simulink model "Newton_Euler_RP_LATEST"  (R2023b)
settings: Solver=VariableStepAuto  StartTime=0.0  StopTime=20  RelTol=1e-3
undefined symbols (not defined in the file or in its folder): L11, L22, M1, M2, X, Y, Z
libraries: nesl_utility x25, sm_lib x20, robotcorelib x1, simulink x1
settings Model: Creator=manu  LastModifiedBy=hdelala
settings DebuggingCC: UnconnectedInputMsg=warning  UnconnectedOutputMsg=warning  UnconnectedLineMsg=warning
settings ModelReferenceCC: EnableRefExpFcnMdlSchedulingChecks=on
settings RTWCC: DLArmComputeVersion=19.05

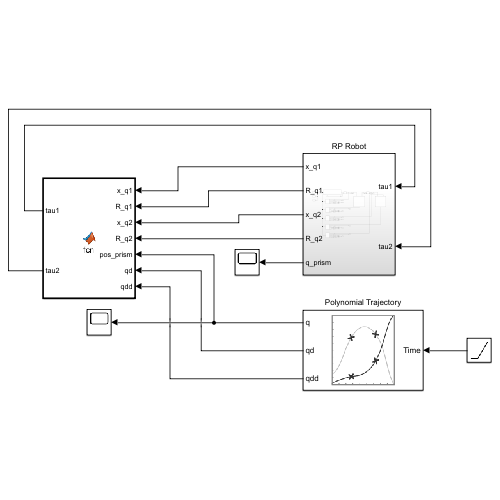
[thumbnail: Simulink's stored preview of the top-level diagram]
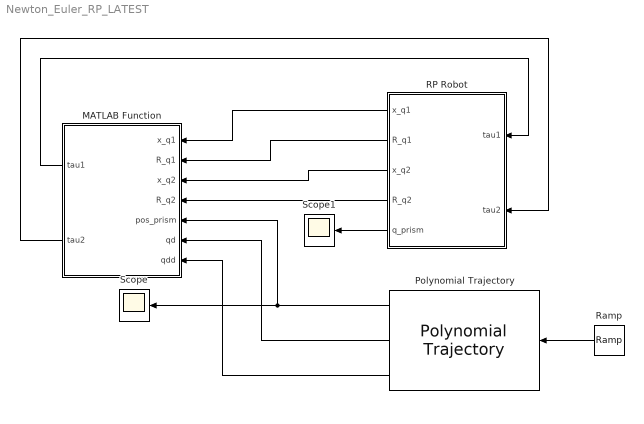
== system Newton_Euler_RP_LATEST ==
  MATLAB Function : MATLAB Function  TreatAsAtomicUnit=on
  Polynomial Trajectory : robotcorelib/Polynomial Trajectory  WaypointSource=Internal  Waypoints=[0,pi/4;-5/100,-10/100]  TimePoints=[ 0, 15 ]  TimeInterval=[ 1, 4 ]  Method=Cubic Polynomial  ParameterSource=Internal  VelocityBoundaryCondition=zeros( 2, 2 )  AccelerationBoundaryCondition=zeros( 2, 5 )  SimulateUsing=Interpreted execution
  RP Robot : Subsystem
  Ramp : simulink/Sources/Ramp  slope=1  start=0  InitialOutput=0
  Scope : Scope
  Scope1 : Scope
  wires:
  Polynomial Trajectory/1 -> MATLAB Function/5(pos_prism), Scope/1
  Ramp/1 -> Polynomial Trajectory/1
  MATLAB Function/2(tau2) -> RP Robot/2(tau2)
  MATLAB Function/1(tau1) -> RP Robot/1(tau1)
  RP Robot/1(x_q1) -> MATLAB Function/1(x_q1)
  RP Robot/2(R_q1) -> MATLAB Function/2(R_q1)
  RP Robot/3(x_q2) -> MATLAB Function/3(x_q2)
  RP Robot/4(R_q2) -> MATLAB Function/4(R_q2)
  Polynomial Trajectory/2 -> MATLAB Function/6(qd)
  Polynomial Trajectory/3 -> MATLAB Function/7(qdd)
  RP Robot/5(q_prism) -> Scope1/1

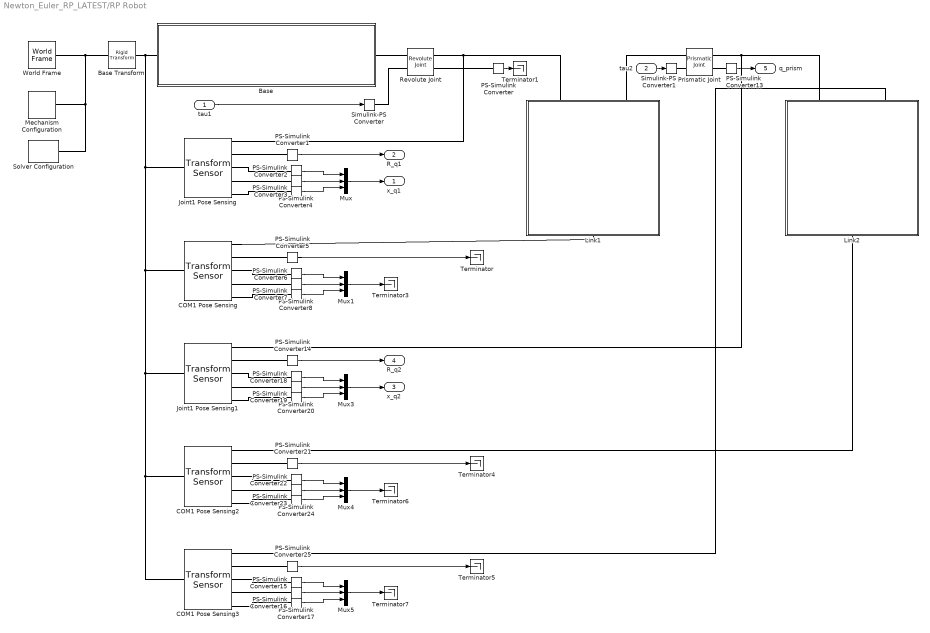
== system Newton_Euler_RP_LATEST/RP Robot ==
  tau1 : Inport
  tau2 : Inport  Port=2
  Base : Subsystem
  Base Transform : sm_lib/Frames and Transforms/Rigid Transform  TranslationMethod=None  TranslationStandardOffset=0  TranslationStandardOffsetUnits=m  TranslationStandardAxis=+Z  TranslationCartesianOffset=[0 0 0]  TranslationCartesianOffsetUnits=m  TranslationROffset=0  TranslationROffsetUnits=m  TranslationZOffset=0  TranslationZOffsetUnits=m  TranslationThetaOffset=0  TranslationThetaOffsetUnits=deg  RotationMethod=AlignedAxes  RotationAngleUnits=deg  RotationStandardAxis=+Z  RotationAngle=0.0  RotationArbitraryAxis=[0 0 1]  FollAlignAxisA=+Z  BaseAlignAxisA=-Y  FollAlignAxisB=+X  BaseAlignAxisB=+X  RotationSequenceAxes=FollowerAxes  RotationSequence=XYX  RotationSequenceAngles=[0 0 0]  RotationSequenceAnglesUnits=deg  RotationMatrix=[1 0 0; 0 1 0; 0 0 1]  Quaternion=[1 0 0 0]
  COM1 Pose Sensing : sm_lib/Frames and Transforms/Transform Sensor  MeasurementFrame=Base  RotationSequence=XYX  SenseAngle=off  SenseAxis=off  SenseQ=off  SenseR=on  SenseRotationSequence=off  SenseOmegaX=off  SenseOmegaY=off  SenseOmegaZ=off  SenseOmega=off  SenseQDot=off  SenseRDot=off  SenseRotationSequenceDot=off  SenseAlphaX=off  SenseAlphaY=off  SenseAlphaZ=off  SenseAlpha=off  SenseQDDot=off  SenseRDDot=off  SenseX=on  SenseY=on  SenseZ=on  SenseXYZ=off  SenseRad=off  SenseAzim=off  SenseDist=off  SenseInc=off  SenseXDot=off  SenseYDot=off  SenseZDot=off  SenseXYZDot=off  SenseRadDot=off  SenseAzimDot=off  SenseDistDot=off  SenseIncDot=off  SenseXDDot=off  SenseYDDot=off  SenseZDDot=off  SenseXYZDDot=off  SenseRadDDot=off  SenseAzimDDot=off  SenseDistDDot=off  SenseIncDDot=off
  COM1 Pose Sensing2 : sm_lib/Frames and Transforms/Transform Sensor  MeasurementFrame=Base  RotationSequence=XYX  SenseAngle=off  SenseAxis=off  SenseQ=off  SenseR=on  SenseRotationSequence=off  SenseOmegaX=off  SenseOmegaY=off  SenseOmegaZ=off  SenseOmega=off  SenseQDot=off  SenseRDot=off  SenseRotationSequenceDot=off  SenseAlphaX=off  SenseAlphaY=off  SenseAlphaZ=off  SenseAlpha=off  SenseQDDot=off  SenseRDDot=off  SenseX=on  SenseY=on  SenseZ=on  SenseXYZ=off  SenseRad=off  SenseAzim=off  SenseDist=off  SenseInc=off  SenseXDot=off  SenseYDot=off  SenseZDot=off  SenseXYZDot=off  SenseRadDot=off  SenseAzimDot=off  SenseDistDot=off  SenseIncDot=off  SenseXDDot=off  SenseYDDot=off  SenseZDDot=off  SenseXYZDDot=off  SenseRadDDot=off  SenseAzimDDot=off  SenseDistDDot=off  SenseIncDDot=off
  COM1 Pose Sensing3 : sm_lib/Frames and Transforms/Transform Sensor  MeasurementFrame=Base  RotationSequence=XYX  SenseAngle=off  SenseAxis=off  SenseQ=off  SenseR=on  SenseRotationSequence=off  SenseOmegaX=off  SenseOmegaY=off  SenseOmegaZ=off  SenseOmega=off  SenseQDot=off  SenseRDot=off  SenseRotationSequenceDot=off  SenseAlphaX=off  SenseAlphaY=off  SenseAlphaZ=off  SenseAlpha=off  SenseQDDot=off  SenseRDDot=off  SenseX=on  SenseY=on  SenseZ=on  SenseXYZ=off  SenseRad=off  SenseAzim=off  SenseDist=off  SenseInc=off  SenseXDot=off  SenseYDot=off  SenseZDot=off  SenseXYZDot=off  SenseRadDot=off  SenseAzimDot=off  SenseDistDot=off  SenseIncDot=off  SenseXDDot=off  SenseYDDot=off  SenseZDDot=off  SenseXYZDDot=off  SenseRadDDot=off  SenseAzimDDot=off  SenseDistDDot=off  SenseIncDDot=off
  Joint1 Pose Sensing : sm_lib/Frames and Transforms/Transform Sensor  MeasurementFrame=Base  RotationSequence=XYX  SenseAngle=off  SenseAxis=off  SenseQ=off  SenseR=on  SenseRotationSequence=off  SenseOmegaX=off  SenseOmegaY=off  SenseOmegaZ=off  SenseOmega=off  SenseQDot=off  SenseRDot=off  SenseRotationSequenceDot=off  SenseAlphaX=off  SenseAlphaY=off  SenseAlphaZ=off  SenseAlpha=off  SenseQDDot=off  SenseRDDot=off  SenseX=on  SenseY=on  SenseZ=on  SenseXYZ=off  SenseRad=off  SenseAzim=off  SenseDist=off  SenseInc=off  SenseXDot=off  SenseYDot=off  SenseZDot=off  SenseXYZDot=off  SenseRadDot=off  SenseAzimDot=off  SenseDistDot=off  SenseIncDot=off  SenseXDDot=off  SenseYDDot=off  SenseZDDot=off  SenseXYZDDot=off  SenseRadDDot=off  SenseAzimDDot=off  SenseDistDDot=off  SenseIncDDot=off
  Joint1 Pose Sensing1 : sm_lib/Frames and Transforms/Transform Sensor  MeasurementFrame=Base  RotationSequence=XYX  SenseAngle=off  SenseAxis=off  SenseQ=off  SenseR=on  SenseRotationSequence=off  SenseOmegaX=off  SenseOmegaY=off  SenseOmegaZ=off  SenseOmega=off  SenseQDot=off  SenseRDot=off  SenseRotationSequenceDot=off  SenseAlphaX=off  SenseAlphaY=off  SenseAlphaZ=off  SenseAlpha=off  SenseQDDot=off  SenseRDDot=off  SenseX=on  SenseY=on  SenseZ=on  SenseXYZ=off  SenseRad=off  SenseAzim=off  SenseDist=off  SenseInc=off  SenseXDot=off  SenseYDot=off  SenseZDot=off  SenseXYZDot=off  SenseRadDot=off  SenseAzimDot=off  SenseDistDot=off  SenseIncDot=off  SenseXDDot=off  SenseYDDot=off  SenseZDDot=off  SenseXYZDDot=off  SenseRadDDot=off  SenseAzimDDot=off  SenseDistDDot=off  SenseIncDDot=off
  Link1 : Subsystem
  Link2 : Subsystem
  Mechanism Configuration : sm_lib/Utilities/Mechanism Configuration  UniformGravity=Constant  GravityVector=[0 0 -9.81]  GravityVectorUnits=m/s^2  LinearizationDelta=0.001  JointModeTransitionNonlinearIterations=2
  Mux{,1,3..5} (5 alike) : Mux  Inputs=3
  PS-Simulink Converter{,1..8,13..25} (22 alike) : nesl_utility/PS-Simulink Converter  PhysicalDomain=network_engine_domain  SubClassName=ps_output  LeftPortType=input  RightPortType=output  PseudoPeriodic=off  Frequencies=[]  VectorFormat=1-D array  Unit=inherit  AffineConversion=off
  Prismatic Joint : sm_lib/Joints/Prismatic Joint  JointMode=Normal  SenseConstraintForce=off  SenseConstraintForceX=off  SenseConstraintForceY=off  SenseConstraintForceZ=off  SenseConstraintTorque=off  SenseConstraintTorqueX=off  SenseConstraintTorqueY=off  SenseConstraintTorqueZ=off  SenseTotalForce=off  SenseTotalForceX=off  SenseTotalForceY=off  SenseTotalForceZ=off  SenseTotalTorque=off  SenseTotalTorqueX=off  SenseTotalTorqueY=off  SenseTotalTorqueZ=off  CompositeWrenchDir=FollowerOnBase  CompositeWrenchFrame=BaseFrame  EquilibriumPosition=0  EquilibriumPositionUnits=m  SpringStiffness=0  SpringStiffnessUnits=N/m  DampingCoefficient=0  DampingCoefficientUnits=N/(m/s)  TorqueActuationMode=InputTorque  MotionActuationMode=ComputedMotion  SensePosition=on  SenseVelocity=off  SenseAcceleration=off  SenseTorqueForce=off  SenseLowerLimitTorqueForce=off  SenseUpperLimitTorqueForce=off  LowerLimitSpecify=off  LowerLimitBound=-25/2  LowerLimitBoundUnits=cm  LowerLimitStiffness=1e6  LowerLimitStiffnessUnits=N/m  LowerLimitDamping=1e3  LowerLimitDampingUnits=N/(m/s)  LowerLimitTransitionRegionWidth=1e-4  LowerLimitTransitionRegionWidthUnits=m  UpperLimitSpecify=off  UpperLimitBound=0  UpperLimitBoundUnits=cm  UpperLimitStiffness=1e6  UpperLimitStiffnessUnits=N/m  UpperLimitDamping=1e3  UpperLimitDampingUnits=N/(m/s)  UpperLimitTransitionRegionWidth=1e-4  UpperLimitTransitionRegionWidthUnits=m  PositionTargetSpecify=on  PositionTargetPriority=High  PositionTargetValue=Q2  PositionTargetValueUnits=cm  VelocityTargetSpecify=off  VelocityTargetPriority=High  VelocityTargetValue=0  VelocityTargetValueUnits=m/s
  Revolute Joint : sm_lib/Joints/Revolute Joint  JointMode=Normal  SenseConstraintForce=off  SenseConstraintForceX=off  SenseConstraintForceY=off  SenseConstraintForceZ=off  SenseConstraintTorque=off  SenseConstraintTorqueX=off  SenseConstraintTorqueY=off  SenseConstraintTorqueZ=off  SenseTotalForce=off  SenseTotalForceX=off  SenseTotalForceY=off  SenseTotalForceZ=off  SenseTotalTorque=off  SenseTotalTorqueX=off  SenseTotalTorqueY=off  SenseTotalTorqueZ=off  CompositeWrenchDir=FollowerOnBase  CompositeWrenchFrame=BaseFrame  EquilibriumPosition=0  EquilibriumPositionUnits=rad  SpringStiffness=0  SpringStiffnessUnits=N*m/rad  DampingCoefficient=0.002  DampingCoefficientUnits=N*m/(rad/s)  TorqueActuationMode=InputTorque  MotionActuationMode=ComputedMotion  SensePosition=on  SenseVelocity=off  SenseAcceleration=off  SenseTorqueForce=off  SenseLowerLimitTorqueForce=off  SenseUpperLimitTorqueForce=off  LowerLimitSpecify=off  LowerLimitBound=-90  LowerLimitBoundUnits=deg  LowerLimitStiffness=1e4  LowerLimitStiffnessUnits=N*m/deg  LowerLimitDamping=10  LowerLimitDampingUnits=N*m/(deg/s)  LowerLimitTransitionRegionWidth=0.1  LowerLimitTransitionRegionWidthUnits=deg  UpperLimitSpecify=off  UpperLimitBound=90  UpperLimitBoundUnits=deg  UpperLimitStiffness=1e4  UpperLimitStiffnessUnits=N*m/deg  UpperLimitDamping=10  UpperLimitDampingUnits=N*m/(deg/s)  UpperLimitTransitionRegionWidth=0.1  UpperLimitTransitionRegionWidthUnits=deg  PositionTargetSpecify=on  PositionTargetPriority=High  PositionTargetValue=Q1  PositionTargetValueUnits=deg  VelocityTargetSpecify=off  VelocityTargetPriority=High  VelocityTargetValue=0  VelocityTargetValueUnits=deg/s
  Simulink-PS Converter : nesl_utility/Simulink-PS Converter  PhysicalDomain=network_engine_domain  SubClassName=ps_input  LeftPortType=input  RightPortType=output  PseudoPeriodic=off  Frequencies=[]  NoiseDistribution=none  NoiseParameters=[]  Unit=1  AffineConversion=off  FilteringAndDerivatives=provide  SimscapeFilterOrder=1  InputFilterTimeConstant=0.001  UdotUserProvided=0
  Simulink-PS Converter1 : nesl_utility/Simulink-PS Converter  PhysicalDomain=network_engine_domain  SubClassName=ps_input  LeftPortType=input  RightPortType=output  PseudoPeriodic=off  Frequencies=[]  NoiseDistribution=none  NoiseParameters=[]  Unit=1  AffineConversion=off  FilteringAndDerivatives=provide  SimscapeFilterOrder=1  InputFilterTimeConstant=0.001  UdotUserProvided=0
  Solver Configuration : nesl_utility/Solver Configuration  PhysicalDomain=network_engine_domain  SubClassName=solver  LeftPortType=input  RightPortType=generic  Tones=[]  Harmonics=[]  SimulateNoise=off  Profile=off  UseLocalSampling=off  EnableSwitchedLinearOptims=on  FrequencyDomain=off  UseCCode=off  RelTol=0.001  AbsTol=1e-06  MinStep=1e-09  ToWorkspace=off  RevertToSquareIcSolve=off  NumHomotopyIterations=100  PhasorMode=off  PhasorModeNumHarmonics=1  ConsistencySolver=NEWTON_FTOL  IndexReductionMethod=DerivativeReplacement  DoDC=off  ResidualTolerance=1e-09  ConsistencyTolSource=GLOBAL  ConsistencyAbsTol=0.001  ConsistencyRelTol=0.001  ConsistencyTolFactor=0.001  UseLocalSolver=off  LocalSolverChoice=NE_BACKWARD_EULER_ADVANCER  ResolveIndetEquations=on  FunctionEvalNumThread=1  LocalSolverSampleTime=0.001  DoFixedCost=off  MaxNonlinIter=3  MaxModeIter=2  ComputeImpulses=off  ImpulseIterations=2  LinearAlgebra=Sparse  LinearAlgebraNumThread=0  EquationFormulation=NE_TIME_EF  DelaysMemoryBudget=1024  AutomaticFiltering=on  FilteringTimeConstant=0.001  PartitionStorageMethod=AS_NEEDED  PartitionMemoryBudget=1024  PartitionMethod=ROBUST  MultibodyUseLocalSolver=off  MultibodyLocalSolverChoice=ODE1  MultibodyLocalSolverSampleTime=0.001
  Terminator{,1,3..7} (7 alike) : Terminator
  World Frame : sm_lib/Frames and Transforms/World Frame
  x_q1 : Outport
  R_q1 : Outport  Port=2
  x_q2 : Outport  Port=3
  R_q2 : Outport  Port=4
  q_prism : Outport  Port=5
  wires:
  PS-Simulink Converter5/1 -> Terminator/1
  Mux1/1 -> Terminator3/1
  PS-Simulink Converter8/1 -> Mux1/2
  PS-Simulink Converter7/1 -> Mux1/3
  PS-Simulink Converter1/1 -> R_q1/1
  PS-Simulink Converter6/1 -> Mux1/1
  PS-Simulink Converter/1 -> Terminator1/1
  PS-Simulink Converter3/1 -> Mux/3
  Mux/1 -> x_q1/1
  tau1/1 -> Simulink-PS Converter/1
  PS-Simulink Converter2/1 -> Mux/1
  PS-Simulink Converter4/1 -> Mux/2
  tau2/1 -> Simulink-PS Converter1/1
  PS-Simulink Converter13/1 -> q_prism/1
  PS-Simulink Converter25/1 -> Terminator5/1
  PS-Simulink Converter15/1 -> Mux5/1
  PS-Simulink Converter17/1 -> Mux5/2
  PS-Simulink Converter16/1 -> Mux5/3
  Mux3/1 -> x_q2/1
  PS-Simulink Converter18/1 -> Mux3/1
  Mux4/1 -> Terminator6/1
  PS-Simulink Converter20/1 -> Mux3/2
  Mux5/1 -> Terminator7/1
  PS-Simulink Converter21/1 -> Terminator4/1
  PS-Simulink Converter23/1 -> Mux4/3
  PS-Simulink Converter14/1 -> R_q2/1
  PS-Simulink Converter24/1 -> Mux4/2
  PS-Simulink Converter19/1 -> Mux3/3
  PS-Simulink Converter22/1 -> Mux4/1
  connections:
  Revolute Joint/RConn2 -- PS-Simulink Converter/LConn1
  Revolute Joint/LConn1 -- Base/RConn1
  COM1 Pose Sensing/RConn4 -- PS-Simulink Converter8/LConn1
  COM1 Pose Sensing/RConn3 -- PS-Simulink Converter6/LConn1
  COM1 Pose Sensing/RConn2 -- PS-Simulink Converter5/LConn1
  Joint1 Pose Sensing1/LConn1 -- COM1 Pose Sensing3/LConn1 -- COM1 Pose Sensing2/LConn1 -- COM1 Pose Sensing/LConn1 -- Joint1 Pose Sensing/LConn1 -- Base Transform/RConn1 -- Base/LConn1
  PS-Simulink Converter1/LConn1 -- Joint1 Pose Sensing/RConn2
  PS-Simulink Converter3/LConn1 -- Joint1 Pose Sensing/RConn5
  Link1/LConn1 -- Joint1 Pose Sensing/RConn1 -- Revolute Joint/RConn1
  Mechanism Configuration/RConn1 -- Base Transform/LConn1 -- World Frame/RConn1 -- Solver Configuration/RConn1
  PS-Simulink Converter4/LConn1 -- Joint1 Pose Sensing/RConn4
  COM1 Pose Sensing/RConn5 -- PS-Simulink Converter7/LConn1
  Simulink-PS Converter/RConn1 -- Revolute Joint/LConn2
  Joint1 Pose Sensing/RConn3 -- PS-Simulink Converter2/LConn1
  COM1 Pose Sensing/RConn1 -- Link1/RConn1
  Link1/LConn2 -- Prismatic Joint/LConn1
  Joint1 Pose Sensing1/RConn1 -- Prismatic Joint/RConn1 -- Link2/LConn1
  Prismatic Joint/LConn2 -- Simulink-PS Converter1/RConn1
  Prismatic Joint/RConn2 -- PS-Simulink Converter13/LConn1
  COM1 Pose Sensing3/RConn5 -- PS-Simulink Converter16/LConn1
  PS-Simulink Converter19/LConn1 -- Joint1 Pose Sensing1/RConn5
  COM1 Pose Sensing3/RConn2 -- PS-Simulink Converter25/LConn1
  COM1 Pose Sensing3/RConn3 -- PS-Simulink Converter15/LConn1
  PS-Simulink Converter20/LConn1 -- Joint1 Pose Sensing1/RConn4
  Joint1 Pose Sensing1/RConn3 -- PS-Simulink Converter18/LConn1
  PS-Simulink Converter14/LConn1 -- Joint1 Pose Sensing1/RConn2
  COM1 Pose Sensing2/RConn2 -- PS-Simulink Converter21/LConn1
  COM1 Pose Sensing2/RConn3 -- PS-Simulink Converter22/LConn1
  COM1 Pose Sensing3/RConn4 -- PS-Simulink Converter17/LConn1
  COM1 Pose Sensing2/RConn5 -- PS-Simulink Converter23/LConn1
  COM1 Pose Sensing2/RConn4 -- PS-Simulink Converter24/LConn1
  Link2/RConn1 -- COM1 Pose Sensing2/RConn1
  COM1 Pose Sensing3/RConn1 -- Link2/LConn2

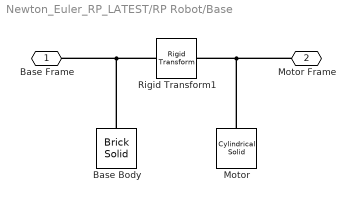
== system Newton_Euler_RP_LATEST/RP Robot/Base ==
  Base Body : sm_lib/Body Elements/Brick Solid  GraphicAmbientColor=[0.15 0.15 0.15 1.0]  BasedOnType=Density  BrickDimensions=[20 20 5]  BrickDimensionsUnits=cm  CenterOfMass=[0 0 0]  CenterOfMassUnits=m  GraphicDiffuseColor=[0.5 0.5 0.5]  Density=1000  DensityUnits=kg/m^3  DoExposeReferenceFrame=on  GraphicEmissiveColor=[0.0 0.0 0.0 1.0]  ExportEntireGeometry=off  SerializedFrames=<Frames/>  MarkerShape=Sphere  MarkerSize=10  GraphicType=FromGeometry  InertiaType=CalculateFromGeometry  Mass=1  MassUnits=kg  MomentsOfInertia=[1 1 1]  MomentsOfInertiaUnits=kg*m^2  GraphicOpacity=1.0  ProductsOfInertia=[0 0 0]  ProductsOfInertiaUnits=kg*m^2  GraphicShininess=75  GraphicSpecularColor=[0.5 0.5 0.5 1.0]  GraphicVisPropType=SimpleVisualProperties
  Motor : sm_lib/Body Elements/Cylindrical Solid  GraphicAmbientColor=[0.15 0.15 0.15 1.0]  BasedOnType=Density  CenterOfMass=[0 0 0]  CenterOfMassUnits=m  GraphicDiffuseColor=[0.0 0.0 0.0]  CylinderLength=5  CylinderLengthUnits=cm  CylinderRadius=3  CylinderRadiusUnits=cm  Density=1000  DensityUnits=kg/m^3  DoExposeReferenceFrame=on  GraphicEmissiveColor=[0.0 0.0 0.0 1.0]  ExportEntireGeometry=off  SerializedFrames=<Frames/>  MarkerShape=Sphere  MarkerSize=10  GraphicType=FromGeometry  InertiaType=CalculateFromGeometry  Mass=1  MassUnits=kg  MomentsOfInertia=[1 1 1]  MomentsOfInertiaUnits=kg*m^2  GraphicOpacity=1.0  ProductsOfInertia=[0 0 0]  ProductsOfInertiaUnits=kg*m^2  GraphicShininess=75  GraphicSpecularColor=[0.5 0.5 0.5 1.0]  GraphicVisPropType=SimpleVisualProperties
  Rigid Transform1 : sm_lib/Frames and Transforms/Rigid Transform  TranslationMethod=StandardAxis  TranslationStandardOffset=5  TranslationStandardOffsetUnits=cm  TranslationStandardAxis=+Z  TranslationCartesianOffset=[0 0 0]  TranslationCartesianOffsetUnits=m  TranslationROffset=0  TranslationROffsetUnits=m  TranslationZOffset=0  TranslationZOffsetUnits=m  TranslationThetaOffset=0  TranslationThetaOffsetUnits=deg  RotationMethod=None  RotationAngleUnits=deg  RotationStandardAxis=+Y  RotationAngle=90  RotationArbitraryAxis=[0 0 1]  FollAlignAxisA=+X  BaseAlignAxisA=+Y  FollAlignAxisB=+Y  BaseAlignAxisB=+Z  RotationSequenceAxes=FollowerAxes  RotationSequence=XYX  RotationSequenceAngles=[0 0 0]  RotationSequenceAnglesUnits=deg  RotationMatrix=[1 0 0; 0 1 0; 0 0 1]  Quaternion=[1 0 0 0]
  Base Frame : PMIOPort  Side=Left
  Motor Frame : PMIOPort  Port=2  Side=Right
  connections:
  Base Body/RConn1 -- Base Frame/RConn1 -- Rigid Transform1/LConn1
  Motor/RConn1 -- Motor Frame/RConn1 -- Rigid Transform1/RConn1

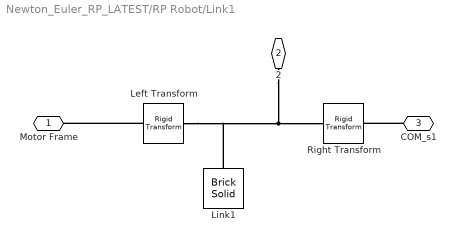
== system Newton_Euler_RP_LATEST/RP Robot/Link1 ==
  Left Transform : sm_lib/Frames and Transforms/Rigid Transform  TranslationMethod=StandardAxis  TranslationStandardOffset=L11/2  TranslationStandardOffsetUnits=cm  TranslationStandardAxis=-X  TranslationCartesianOffset=[0.7 0.5 0]  TranslationCartesianOffsetUnits=m  TranslationROffset=0  TranslationROffsetUnits=m  TranslationZOffset=0  TranslationZOffsetUnits=m  TranslationThetaOffset=0  TranslationThetaOffsetUnits=deg  RotationMethod=None  RotationAngleUnits=deg  RotationStandardAxis=+Y  RotationAngle=90  RotationArbitraryAxis=[0 0 1]  FollAlignAxisA=+X  BaseAlignAxisA=+Y  FollAlignAxisB=+Y  BaseAlignAxisB=+Z  RotationSequenceAxes=FollowerAxes  RotationSequence=XYX  RotationSequenceAngles=[0 0 0]  RotationSequenceAnglesUnits=deg  RotationMatrix=[1 0 0; 0 1 0; 0 0 1]  Quaternion=[1 0 0 0]
  Link1 : sm_lib/Body Elements/Brick Solid  GraphicAmbientColor=[0.15 0.15 0.15 1.0]  BasedOnType=Mass  BrickDimensions=[L11 3 3]  BrickDimensionsUnits=cm  CenterOfMass=[0 0 0]  CenterOfMassUnits=m  GraphicDiffuseColor=[1.0 0.0 0.0]  Density=1000  DensityUnits=kg/m^3  DoExposeReferenceFrame=on  GraphicEmissiveColor=[0.0 0.0 0.0 1.0]  ExportEntireGeometry=off  SerializedFrames=<Frames/>  MarkerShape=Sphere  MarkerSize=10  GraphicType=FromGeometry  InertiaType=CalculateFromGeometry  Mass=M1  MassUnits=kg  MomentsOfInertia=[1 1 1]  MomentsOfInertiaUnits=kg*m^2  GraphicOpacity=1.0  ProductsOfInertia=[0 0 0]  ProductsOfInertiaUnits=kg*m^2  GraphicShininess=75  GraphicSpecularColor=[0.5 0.5 0.5 1.0]  GraphicVisPropType=SimpleVisualProperties
  Right Transform : sm_lib/Frames and Transforms/Rigid Transform  TranslationMethod=StandardAxis  TranslationStandardOffset=L11/2  TranslationStandardOffsetUnits=cm  TranslationStandardAxis=+X  TranslationCartesianOffset=[0 0 0]  TranslationCartesianOffsetUnits=m  TranslationROffset=0  TranslationROffsetUnits=m  TranslationZOffset=0  TranslationZOffsetUnits=m  TranslationThetaOffset=0  TranslationThetaOffsetUnits=deg  RotationMethod=AlignedAxes  RotationAngleUnits=deg  RotationStandardAxis=+Z  RotationAngle=0.0  RotationArbitraryAxis=[0 0 1]  FollAlignAxisA=+Z  BaseAlignAxisA=+X  FollAlignAxisB=+Y  BaseAlignAxisB=+Y  RotationSequenceAxes=FollowerAxes  RotationSequence=XYX  RotationSequenceAngles=[0 0 0]  RotationSequenceAnglesUnits=deg  RotationMatrix=[1 0 0; 0 1 0; 0 0 1]  Quaternion=[1 0 0 0]
  Motor Frame : PMIOPort  Side=Left
  2 : PMIOPort  Port=2  Side=Right
  COM_s1 : PMIOPort  Port=3  Side=Left
  connections:
  2/RConn1 -- Left Transform/LConn1 -- Link1/RConn1 -- Right Transform/LConn1
  COM_s1/RConn1 -- Right Transform/RConn1
  Left Transform/RConn1 -- Motor Frame/RConn1

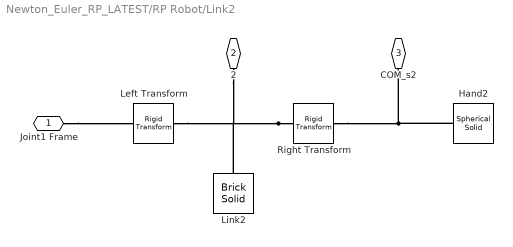
== system Newton_Euler_RP_LATEST/RP Robot/Link2 ==
  Hand2 : sm_lib/Body Elements/Spherical Solid  GraphicAmbientColor=[0.15 0.15 0.15 1.0]  BasedOnType=Mass  CenterOfMass=[0 0 0]  CenterOfMassUnits=m  GraphicDiffuseColor=[0.2 0.2 1.0]  Density=1000  DensityUnits=kg/m^3  DoExposeReferenceFrame=on  GraphicEmissiveColor=[0.0 0.0 0.0 1.0]  ExportEntireGeometry=off  SerializedExposedGeometries=<exposedGeometries/>  SerializedFrames=<Frames/>  MarkerShape=Sphere  MarkerSize=10  GraphicType=FromGeometry  InertiaType=CalculateFromGeometry  Mass=0  MassUnits=kg  MomentsOfInertia=[1 1 1]  MomentsOfInertiaUnits=kg*m^2  GraphicOpacity=1.0  ProductsOfInertia=[0 0 0]  ProductsOfInertiaUnits=kg*m^2  GraphicShininess=75  GraphicSpecularColor=[0.5 0.5 0.5 1.0]  SphereRadius=3  SphereRadiusUnits=cm  GraphicVisPropType=SimpleVisualProperties
  Left Transform : sm_lib/Frames and Transforms/Rigid Transform  TranslationMethod=StandardAxis  TranslationStandardOffset=L22/2  TranslationStandardOffsetUnits=cm  TranslationStandardAxis=-X  TranslationCartesianOffset=[0.7 0.5 0]  TranslationCartesianOffsetUnits=m  TranslationROffset=0  TranslationROffsetUnits=m  TranslationZOffset=0  TranslationZOffsetUnits=m  TranslationThetaOffset=0  TranslationThetaOffsetUnits=deg  RotationMethod=StandardAxis  RotationAngleUnits=deg  RotationStandardAxis=+Y  RotationAngle=90  RotationArbitraryAxis=[0 0 1]  FollAlignAxisA=+X  BaseAlignAxisA=+Y  FollAlignAxisB=+Y  BaseAlignAxisB=+Z  RotationSequenceAxes=FollowerAxes  RotationSequence=XYX  RotationSequenceAngles=[0 0 0]  RotationSequenceAnglesUnits=deg  RotationMatrix=[1 0 0; 0 1 0; 0 0 1]  Quaternion=[1 0 0 0]
  Link2 : sm_lib/Body Elements/Brick Solid  GraphicAmbientColor=[0.15 0.15 0.15 1.0]  BasedOnType=Mass  BrickDimensions=[L22 2 2]  BrickDimensionsUnits=cm  CenterOfMass=[0 0 0]  CenterOfMassUnits=m  GraphicDiffuseColor=[1.0 0.0 0.0]  Density=1000  DensityUnits=kg/m^3  DoExposeReferenceFrame=on  GraphicEmissiveColor=[0.0 0.0 0.0 1.0]  ExportEntireGeometry=off  SerializedFrames=<Frames/>  MarkerShape=Sphere  MarkerSize=10  GraphicType=FromGeometry  InertiaType=CalculateFromGeometry  Mass=M2  MassUnits=kg  MomentsOfInertia=[1 1 1]  MomentsOfInertiaUnits=kg*m^2  GraphicOpacity=1.0  ProductsOfInertia=[0 0 0]  ProductsOfInertiaUnits=kg*m^2  GraphicShininess=75  GraphicSpecularColor=[0.5 0.5 0.5 1.0]  GraphicVisPropType=SimpleVisualProperties
  Right Transform : sm_lib/Frames and Transforms/Rigid Transform  TranslationMethod=StandardAxis  TranslationStandardOffset=L22/2  TranslationStandardOffsetUnits=cm  TranslationStandardAxis=+X  TranslationCartesianOffset=[0 0 0]  TranslationCartesianOffsetUnits=m  TranslationROffset=0  TranslationROffsetUnits=m  TranslationZOffset=0  TranslationZOffsetUnits=m  TranslationThetaOffset=0  TranslationThetaOffsetUnits=deg  RotationMethod=None  RotationAngleUnits=deg  RotationStandardAxis=+Z  RotationAngle=0.0  RotationArbitraryAxis=[0 0 1]  FollAlignAxisA=+X  BaseAlignAxisA=+Y  FollAlignAxisB=+Y  BaseAlignAxisB=+Z  RotationSequenceAxes=FollowerAxes  RotationSequence=XYX  RotationSequenceAngles=[0 0 0]  RotationSequenceAnglesUnits=deg  RotationMatrix=[1 0 0; 0 1 0; 0 0 1]  Quaternion=[1 0 0 0]
  Joint1 Frame : PMIOPort  Side=Left
  2 : PMIOPort  Port=2  Side=Right
  COM_s2 : PMIOPort  Port=3  Side=Left
  connections:
  Right Transform/LConn1 -- Link2/RConn1 -- Left Transform/LConn1 -- 2/RConn1
  Hand2/RConn1 -- Right Transform/RConn1 -- COM_s2/RConn1
  Joint1 Frame/RConn1 -- Left Transform/RConn1

== matlab function Newton_Euler_RP_LATEST/MATLAB Function ==
  data: x_q1 input; R_q1 input; x_q2 input; tau1 output; R_q2 input; pos_prism input; tau2 output; qd input; qdd input; M1 parameter; M2 parameter; L11 parameter; L22 parameter
%% This function computes the forward and backward recursion algorithm (Newton-Euler algorithm) for a 2-link robot.
function [tau1, tau2] = fcn(x_q1, R_q1, x_q2, R_q2, pos_prism, qd, qdd, M1, M2, L11, L22)
    %% Initialization

    % Extract joint velocities, accelerations and prismatic joint position
    d_q1=qd(1);
    d_q2=qd(2);
    dd_q1=qdd(1);
    dd_q2=qdd(2);
    %q_prism=pos_prism(2);
    
    % Define robot parameters (Note: link1 is a rotational joints whereas link2 is a translational joint)
    L1 = L11/100; % Lenght of link1 in metres
    L2 = L22/100; % Lenght of link2 in metres
    m1 = M1;      % Mass of the links1 in Kg
    m2 = M2;    % Mass of the links2
    
    % Define inertia matrices for each link
    I1=[1/12*m1*L1^2, 0, 0; 0, 1/12*m1*L1^2, 0; 0, 0, 1/12*m1*L1^2];  
    I2=[1/12*m2*L2^2, 0, 0; 0, 1/12*m2*L2^2, 0; 0, 0, 1/12*m2*L2^2];
    
    % Rotation matrices for joint positions
    R_01=R_q1;       % Rotation matrix of joint1 wrt base frame
    R_02=R_q2;       % Rotation matrix of joint2 wrt base frame
    R_12=R_01'*R_02;
    R_23=eye(3);
    
    % Define position vectors
    P1=x_q1;              % Distance between joint1 and base wrt base
    P2=R_01'*(x_q2-x_q1); % Distance between joint2 and joint1 wrt joint1
    
    % Define positions of the centers of mass (COM)
    Pc1=L1/2*[1;0;0]; % Position of COM1 wrt joint1
    Pc2=L2/2*[0;0;1]; % Position of COM2 wrt joint2

    % Define gravitational acceleration
    g = [0; 9.81; 0]; % Gravity wrt the base
    
    % Assumptions for a fixed base robot
    w0=[0;0;0];
    w0_dot=[0;0;0];
    v0_dot=g;

    % Define rotation axes
    z1=[0;0;1];
    z2=[0;0;1];

    % Initialize forces and torques on the end-effector
    fee=[0;0;0];
    nee=[0;0;0];

    %% FORWARD RECURSIVE ALGORITHM STEPS

    % Step1: Compute Angular Velocity of the two links
    w1=R_01'*w0+d_q1*z1;
    w2=R_12'*w1;

    % Step2: Compute Angular Acceleration of the two links
    w1_dot=R_01'*w0_dot+cross(R_01'*w0, d_q1*z1)+dd_q1*z1;
    w2_dot=R_12'*w1_dot;

    % Step3: Compute Linear Acceleration of the two links 
    v1_dot=R_01'*(cross(w0_dot, P1)+cross(w0, cross(w0, P1))+v0_dot);
    v2_dot=R_12'*(cross(w1_dot, P2)+cross(w1, cross(w1, P2))+v1_dot)+2*cross(R_12'*w1, d_q2*z2)+dd_q2*z2;
    
    % Step4: Compute Linear Acceleration of the COM of the two links
    v1_dot_com=cross(w1_dot, Pc1)+cross(w1, cross(w1, Pc1))+v1_dot;
    v2_dot_com=cross(w2_dot, Pc2)+cross(w2, cross(w2, Pc2))+v2_dot;
   
    % Step5: Compute Forces acting on the COM of the two links 
    F1=m1*v1_dot_com;
    F2=m2*v2_dot_com;

    % Step6: Compute Torques acting about the COM of the two links
    N1=I1*w1_dot+cross(w1, I1*w1);
    N2=I2*w2_dot+cross(w2, I2*w2);
    
    %% BACKWARD RECURSIVE ALGORITHM STEPS

    % Step1: Compute Forces acting on the two joints
    f2=R_23*fee+F2;
    f1=R_12*f2+F1;

    % Step2: Compute Torque acting on the two joints
    n2=N2+R_23*nee+cross(Pc2, F2);
    n1=N1+R_12*n2+cross(Pc1, F1)+cross(P2, R_12*f2);

    % Step3: Compute Torque acting on the two joints motion axis
    tau1=n1'*z1;
    tau2=f2'*z2;
    
end
